simulink model "TheVelocityFuzzyController"  (R2021a)
settings: Solver=VariableStepAuto  StartTime=0.0  StopTime=10.0  RelTol=1e-3
settings Model: Creator=rasm4  LastModifiedBy=rasm4

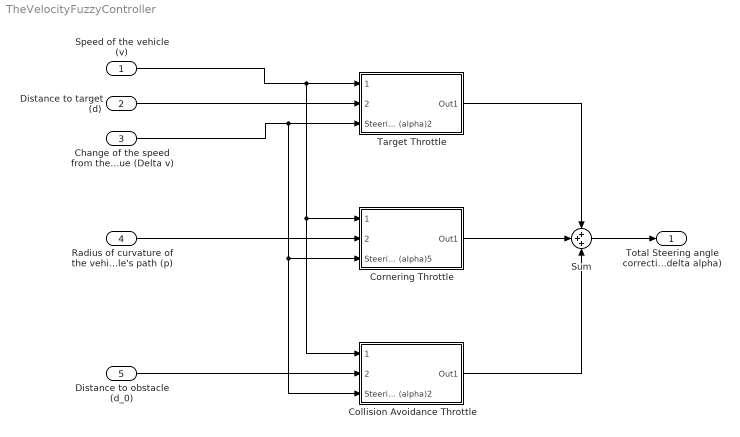
== system TheVelocityFuzzyController ==
  Speed of the vehicle (v) : Inport
  Distance to target (d) : Inport  Port=2
  Change of the speed from the previously measured valcue (Delta v) : Inport  Port=3
  Radius of curvature of the vehicle's path (p) : Inport  Port=4
  Distance to obstacle (d_0) : Inport  Port=5
  Collision Avoidance Throttle : Subsystem
  Cornering Throttle : Subsystem
  Sum : Sum  Inputs=+++
  Target Throttle : Subsystem
  Total Steering angle correction (delta alpha) : Outport
  wires:
  Cornering Throttle/1(Out1) -> Sum/2
  Target Throttle/1(Out1) -> Sum/1
  Collision Avoidance Throttle/1(Out1) -> Sum/3
  Sum/1 -> Total Steering angle correction (delta alpha)/1
  Distance to target (d)/1 -> Target Throttle/2
  Speed of the vehicle (v)/1 -> Cornering Throttle/1, Collision Avoidance Throttle/1, Target Throttle/1
  Radius of curvature of the vehicle's path (p)/1 -> Cornering Throttle/2
  Change of the speed from the previously measured valcue (Delta v)/1 -> Collision Avoidance Throttle/3(Steering angle (alpha)2), Cornering Throttle/3(Steering angle (alpha)5), Target Throttle/3(Steering angle (alpha)2)
  Distance to obstacle (d_0)/1 -> Collision Avoidance Throttle/2

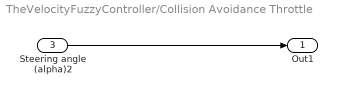
== system TheVelocityFuzzyController/Collision Avoidance Throttle ==
  Steering angle (alpha)2 : Inport  Port=3
  Out1 : Outport
  wires:
  Steering angle (alpha)2/1 -> Out1/1

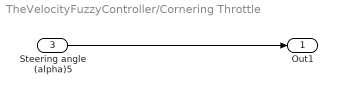
== system TheVelocityFuzzyController/Cornering Throttle ==
  Steering angle (alpha)5 : Inport  Port=3
  Out1 : Outport
  wires:
  Steering angle (alpha)5/1 -> Out1/1

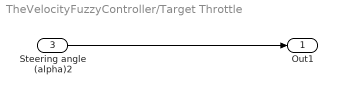
== system TheVelocityFuzzyController/Target Throttle ==
  Steering angle (alpha)2 : Inport  Port=3
  Out1 : Outport
  wires:
  Steering angle (alpha)2/1 -> Out1/1
